simulink model "inverter_with_changing_VDC"  (R2013b)
settings: Solver=ode45  StartTime=0.0  StopTime=T  MaxStep=MaxStep  RelTol=RelTol
values from neighbouring files (symbols this model uses):
  a = b*(Cap*omega)    [it_generator.m]
  b = 0.0123    [it_generator.m]
  c3 = 1*(1+e+e3)    (= 1.11)    [initialization.m]
  Cap = 0.04    [initialization.m]
  ci = 1*(1-e)    (= 0.9)    [initialization.m]
  co = 1*(1+e)    (= 1.1)    [initialization.m]
  J = 2e4    (= 20000)    [initialization.m]
  L = 0.1    [initialization.m]
  R = 0.6    [initialization.m]
  rule = 1    [initialization.m]
  T = 8    [initialization.m]
  x0 = [iL0; vC0; p0;q0]    [initialization.m]
libraries: simulink x3
settings Model: Creator=Amy  LastModifiedBy=Amy

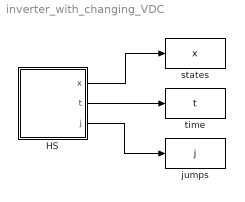
== system inverter_with_changing_VDC ==
  HS : Subsystem  LoadFcn=set_param(gcb,'LinkStatus','none')
      settings: CopyFcn=|
      | set_param(gcb,'LinkStatus','none'),
      | set_param(gcs, 'MaxStep', 'MaxStep', 'RelTol', 'RelTol','Stop time', 'T')
      mask Display:
      | image(imread('Hcal.jpg'))
      | %plot([5 20 20 5 5],[5 5 20 20 5])
      | %text(8,13,'HyEq_mdl')
      | port_label('output', 1, 'x')
      | port_label('output', 2, 't')
      | port_label('output', 3, 'j')
  jumps : ToWorkspace  VariableName=j  SampleTime=-1
  states : ToWorkspace  VariableName=x  SampleTime=-1
  time : ToWorkspace  VariableName=t  SampleTime=-1
  wires:
  HS/1(x) -> states/1
  HS/2(t) -> time/1
  HS/3(j) -> jumps/1

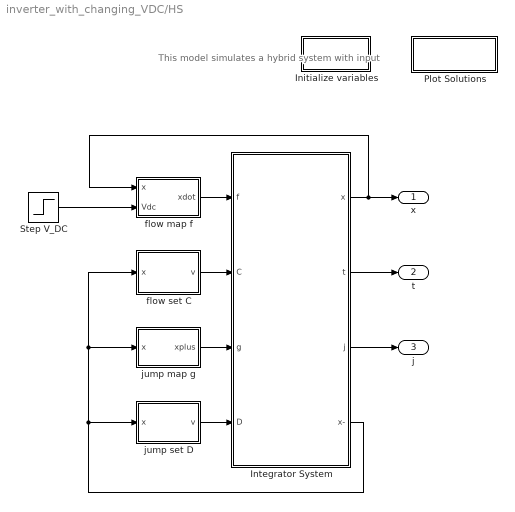
== system inverter_with_changing_VDC/HS ==
  note: This model simulates a hybrid system with input
  Initialize variables : Subsystem  Priority=-10
      settings: OpenFcn=|
      | try
      |      clearvars -except inifile pathfile_in pathfile_pos posfile
      |      cd(pathfile_in);
      |      eval(inifile);
      | catch
      |      [inifile,pathfile_in] = getInitializationfile;
      |      cd(pathfile_in);
      |      inifile = strrep(inifile,'.m','');
      |      eval(inifile);
      | end
      mask Display: disp('Double Click\n to Initialize')
  Integrator System : Subsystem  Priority=2  mask(Hybrid Integrator){T=T, J=J, x0=x0}
      mask prompts: T "Flow Horizon"; J "Jump Horizon"; x0 "Initial Condition"
      mask help:
      | This block integrates the state of the hybrid system defined by the flow map f (first input), the flow set C (second input), the jump map g (third input) and the jump set D (fourth input).
      | Starting from the initial condition x0 (last mask parameter), the system's state x evolves continuously within the set C, according to f(x,u), but is also subject to jumps within D, according to g(x,u).
      | The block also stops the simulation when the time t is greater than the flow horizon T (first mask parameter), or when the number of jumps j is greater than the jump horizon J (second mask parameter).
      | The outputs of the blocks are respectively x(t), t, j, x(t-).
      mask Help:
      | This block integrates the state of the hybrid system defined by the flow map f (first input), the flow set C (second input), the jump map g (third input) and the jump set D (fourth input).
      | <br>
      | Starting from the initial condition x0 (last mask parameter), the system's state x evolves continuously within the set C, according to f(x,u), but is also subject to jumps within D, according to g(x,u).
      | <br>
      | The block also stops the simulation when the time t is greater than the flow horizon T (first mask parameter), or when the number of jumps j is greater than the jump horizon J (second mask parameter).
      | <br>
      | The outputs of the blocks are respectively x(t), t, j, x(t-).
      | <br>
      | You can right click on the block and "Look under mask" to see what's inside the block.
      | Finally, refer to the manual (HybridSimulator_vXX.pdf) for more detailed information on how this hybrid simulator works.
  Plot Solutions : Subsystem
      settings: OpenFcn=|
      | try
      |      cd(pathfile_pos);
      |      eval(posfile);
      | catch
      |      [posfile,pathfile_pos] = getInitializationfile;
      |      cd(pathfile_pos);
      |      posfile = strrep(posfile,'.m','');
      |      eval(posfile);
      | end
      mask Display: disp('Double Click to\n Plot Solutions')
  Step V_DC : Step  Time=3  Before=5  After=7  SampleTime=0
  flow map f : MATLAB Function  TreatAsAtomicUnit=on
  flow set C : MATLAB Function  TreatAsAtomicUnit=on
  jump map g : MATLAB Function  Priority=2  TreatAsAtomicUnit=on
  jump set D : MATLAB Function  TreatAsAtomicUnit=on
  x : Outport
  t : Outport  Port=2
  j : Outport  Port=3
  wires:
  jump map g/1(xplus) -> Integrator System/3(g)
  jump set D/1(v) -> Integrator System/4(D)
  Integrator System/3(j) -> j/1
  Integrator System/2(t) -> t/1
  flow set C/1(v) -> Integrator System/2(C)
  Integrator System/1(x) -> flow map f/1(x), x/1
  Integrator System/4(x-) -> jump set D/1(x), jump map g/1(x), flow set C/1(x)
  flow map f/1(xdot) -> Integrator System/1(f)
  Step V_DC/1 -> flow map f/2(Vdc)

== system inverter_with_changing_VDC/HS/Initialize variables ==

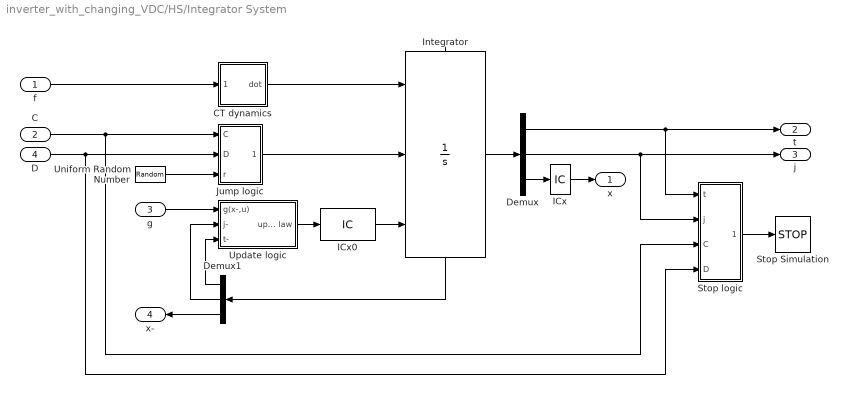
== system inverter_with_changing_VDC/HS/Integrator System ==
  f : Inport
  C : Inport  Port=2
  g : Inport  Port=3
  D : Inport  Port=4
  CT dynamics : Subsystem
  Demux : Demux  Outputs=[1 1 -1]
  Demux1 : Demux  Outputs=[1 1 -1]
  ICx : InitialCondition  Value=x0
  ICx0 : InitialCondition  Value=[0; 0; x0(:)]
  Integrator : Integrator  ExternalReset=level hold  InitialConditionSource=external  ShowStatePort=on  ZeroCross=off
  Jump logic : Subsystem
  Stop Simulation : Stop
  Stop logic : Subsystem
  Uniform Random Number : UniformRandomNumber  Minimum=0  Seed=abs(floor(100*rand))  SampleTime=0
  Update logic : Subsystem
  x : Outport
  t : Outport  Port=2
  j : Outport  Port=3
  x- : Outport  Port=4
  wires:
  ICx0/1 -> Integrator/3
  ICx/1 -> x/1
  Demux/3 -> ICx/1
  Integrator/State -> Demux1/1
  Demux/2 -> j/1, Stop logic/2(j)
  Demux/1 -> t/1, Stop logic/1(t)
  Update logic/1(update law) -> ICx0/1
  CT dynamics/1(dot) -> Integrator/1
  Stop logic/1(stop) -> Stop Simulation/1
  Integrator/1 -> Demux/1
  C/1 -> Stop logic/3(C), Jump logic/1(C)
  D/1 -> Stop logic/4(D), Jump logic/2(D)
  f/1 -> CT dynamics/1(f(x,u))
  Demux1/3 -> x-/1
  Jump logic/1(jump) -> Integrator/2
  Uniform Random Number/1 -> Jump logic/3(r)
  g/1 -> Update logic/1(g(x-,u))
  Demux1/1 -> Update logic/3(t-)
  Demux1/2 -> Update logic/2(j-)

== system inverter_with_changing_VDC/HS/Plot Solutions ==

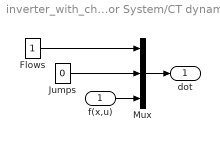
== system inverter_with_changing_VDC/HS/Integrator System/CT dynamics ==
  f(x,u) : Inport
  Flows : Constant
  Jumps : Constant  Value=0
  Mux : Mux  Inputs=[1 1 -1]
  dot : Outport
  wires:
  Jumps/1 -> Mux/2
  Flows/1 -> Mux/1
  Mux/1 -> dot/1
  f(x,u)/1 -> Mux/3

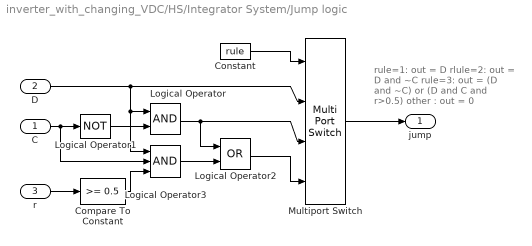
== system inverter_with_changing_VDC/HS/Integrator System/Jump logic ==
  note: rule=1:  out = D
      | rlule=2: out = D and ~C
      | rule=3:  out = (D and ~C)  or (D and C and r>0.5)
      | other :  out = 0
  C : Inport
  D : Inport  Port=2
  r : Inport  Port=3
  Compare To Constant : simulink/Logic and Bit Operations/Compare To Constant  relop=>=  const=0.5  OutDataTypeStr=uint8
  Constant : Constant  Value=rule
  Logical Operator : Logic  AllPortsSameDT=off  OutDataTypeStr=boolean
  Logical Operator1 : Logic  Operator=NOT  Inputs=1  AllPortsSameDT=off  OutDataTypeStr=boolean
  Logical Operator2 : Logic  Operator=OR  AllPortsSameDT=off  OutDataTypeStr=boolean
  Logical Operator3 : Logic  Inputs=3  AllPortsSameDT=off  OutDataTypeStr=boolean
  Multiport Switch : MultiPortSwitch
  jump : Outport
  wires:
  Constant/1 -> Multiport Switch/1
  D/1 -> Logical Operator3/1, Logical Operator/1, Multiport Switch/2
  r/1 -> Compare To Constant/1
  C/1 -> Logical Operator3/2, Logical Operator1/1
  Logical Operator1/1 -> Logical Operator/2
  Logical Operator/1 -> Multiport Switch/3, Logical Operator2/1
  Logical Operator2/1 -> Multiport Switch/4
  Multiport Switch/1 -> jump/1
  Compare To Constant/1 -> Logical Operator3/3
  Logical Operator3/1 -> Logical Operator2/2

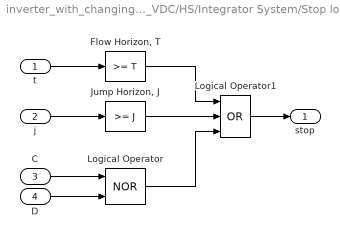
== system inverter_with_changing_VDC/HS/Integrator System/Stop logic ==
  t : Inport
  j : Inport  Port=2
  C : Inport  Port=3
  D : Inport  Port=4
  "Flow Horizon, T" : simulink/Logic and Bit Operations/Compare To Constant  relop=>=  const=T  OutDataTypeStr=uint8  ZeroCross=off
  "Jump Horizon, J" : simulink/Logic and Bit Operations/Compare To Constant  relop=>=  const=J  OutDataTypeStr=uint8  ZeroCross=off
  Logical Operator : Logic  Operator=NOR  AllPortsSameDT=off  OutDataTypeStr=boolean
  Logical Operator1 : Logic  Operator=OR  Inputs=3  AllPortsSameDT=off  OutDataTypeStr=boolean
  stop : Outport
  wires:
  "Flow Horizon, T"/1 -> Logical Operator1/1
  "Jump Horizon, J"/1 -> Logical Operator1/2
  Logical Operator/1 -> Logical Operator1/3
  D/1 -> Logical Operator/2
  t/1 -> "Flow Horizon, T"/1
  j/1 -> "Jump Horizon, J"/1
  C/1 -> Logical Operator/1
  Logical Operator1/1 -> stop/1

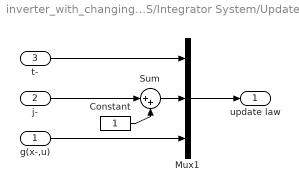
== system inverter_with_changing_VDC/HS/Integrator System/Update logic ==
  g(x-,u) : Inport
  j- : Inport  Port=2
  t- : Inport  Port=3
  Constant : Constant
  Mux1 : Mux  Inputs=[1 1 -1]
  Sum : Sum  Inputs=|++
  update law : Outport
  wires:
  Sum/1 -> Mux1/2
  Mux1/1 -> update law/1
  j-/1 -> Sum/1
  g(x-,u)/1 -> Mux1/3
  t-/1 -> Mux1/1
  Constant/1 -> Sum/2

== matlab function inverter_with_changing_VDC/HS/flow map f ==
  data: x input; xdot output; R parameter; L parameter; Cap parameter; Vdc input
function xdot = f(x, R, L, Cap, Vdc)
%%%%%%%%%%%%%%%%%%%%%%%%%%%%%%%%%%%%%%%%%%%%%%%%%%%%%%%%%%%%%%%%%%%%%%%%%%%
% Matlab M-file       
% Project: DC/AC inverter
%
% Name: f.m
%
% Description: Flow map
%
% Version: v1.8 lite
% Required files: - 
%%%%%%%%%%%%%%%%%%%%%%%%%%%%%%%%%%%%%%%%%%%%%%%%%%%%%%%%%%%%%%%%%%%%%%%%%%%
% states
  iL = x(1);
  vC = x(2);
  p = x(3);
  q = x(4);

% flow map
  iLdot = -R/L*iL - 1/L*vC + Vdc/L*q;
  vCdot = 1/Cap*iL;
  pdot = 0;
  qdot = 0;
  
xdot = [iLdot; vCdot; pdot; qdot];

== matlab function inverter_with_changing_VDC/HS/flow set C ==
  data: x input; v output; a parameter; b parameter; ci parameter; co parameter; c3 parameter; e1 parameter
function v  = C(x, a, b, ci, co, c3, e1) 
%%%%%%%%%%%%%%%%%%%%%%%%%%%%%%%%%%%%%%%%%%%%%%%%%%%%%%%%%%%%%%%%%%%%%%%%%%%
% Matlab M-file       
% Project: DC/AC inverter
%
% Name: C.m
%
% Description: Flow set
%
% Version: v1.8 
% Required files: - 
%%%%%%%%%%%%%%%%%%%%%%%%%%%%%%%%%%%%%%%%%%%%%%%%%%%%%%%%%%%%%%%%%%%%%%%%%%% 
% states
  iL = x(1);
  vC = x(2);
  p = x(3);
  q = x(4);

% useful expressions
  V = (iL/a)^2 + (vC/b)^2;
  qua = quadrant(iL, vC);  
  
% flow set
  if p == 1 
      if V >= ci && V <= co % Hs, Hfw flow
          v = 1;
      elseif q == -1 
          if iL <=0 &&  V <= ci % switch q accroding to Hfw 
              v = 1;
          elseif V >= co && V <= c3 && (qua == 1 || (qua == 4 && iL >= e1))
          % switch q accroding to Hfw
              v = 1;
          else
              v = 0;
          end
      elseif q == 1 
          if iL >=0 && V <= ci % switch q accroding to Hfw 
              v = 1;
          elseif V >= co && V <= c3 && (qua == 3 || (qua == 2 && iL <= -e1)) 
          % switch q accroding to Hfw 
              v = 1;
          else
              v = 0;
          end
      else
          v = 0;          
      end
  elseif p == 2
      if q == 0 && V >= co % Hs, Hg flow
          v = 1;
      elseif (q ~= 0) && V <= ci % Hs, Hg flow
          v = 1;
      else
          v = 0;
      end
  else 
      v = 0;
  end


% if V >= ci && V <= co && p == 1 % Hs, Hfw flow
%      v = 1;
%   elseif V <= ci && p == 1 && q == -1 && iL <=0 
%       % switch q accroding to Hfw 
%      v = 1;
%   elseif V >= co && V <= c3 && p == 1 && q == -1 && (qua == 1 || (qua == 4 && iL >= e1)) 
%       % switch q accroding to Hfw 
%      v = 1;
%   elseif V <= ci && p == 1 && q == 1 && iL >=0 
%       % switch q accroding to Hfw 
%      v = 1;
%   elseif V >= co && V <= c3 && p == 1 && q == 1 && (qua == 3 || (qua == 2 && iL <= -e1)) 
%       % switch q accroding to Hfw 
%      v = 1;
%      
%   elseif V >= co && p == 2 && q == 0 % Hs, Hg flow
%      v = 1;
%   elseif V <= ci && p == 2 && (q == 1 || q == -1) % Hs, Hg flow
%      v = 1;
%   else
%      v = 0;
%   end
% end

== matlab function inverter_with_changing_VDC/HS/jump map g ==
  data: x input; a parameter; b parameter; xplus output; co parameter; ci parameter; c3 parameter; e1 parameter
function xplus = g(x, a, b, co, ci, c3, e1)
%%%%%%%%%%%%%%%%%%%%%%%%%%%%%%%%%%%%%%%%%%%%%%%%%%%%%%%%%%%%%%%%%%%%%%%%%%%
% Matlab M-file       
% Project: DC/AC inverter
%
% Name: g.m
%
% Description: Jump map
%
% Version: v1.8 
% Required files: - 
%%%%%%%%%%%%%%%%%%%%%%%%%%%%%%%%%%%%%%%%%%%%%%%%%%%%%%%%%%%%%%%%%%%%%%%%%%%
% states
  iL = x(1);
  vC = x(2);
  p = x(3);
  q = x(4);  

% useful expressions
  V = (iL/a)^2 + (vC/b)^2;
  qua = quadrant(iL, vC);  
  
% jump map
  iLplus = iL;
  vCplus = vC;
  
  if p == 1
      if q ~= -1 && iL <=0 && V <= ci % switch q accroding to Hfw 
          pplus = p;
          qplus = -1;
      elseif q == 1 && V <= c3 && V >= co && (qua == 1 || (qua == 4 && iL >= e1)) 
      % switch q accroding to Hfw 
          pplus = p;
          qplus = -1;
      elseif V <= c3 && V >= co &&...
          ((qua == 4 && iL <= e1 && q == 1) || (qua == 2 && iL >= -e1 && q == -1))
      % switch q accroding to Hfw
          pplus = p;
          qplus = 0;
      elseif q ~= 1 && iL >=0 && V <= ci
      % switch q accroding to Hfw 
          pplus = p;
          qplus = 1;
      elseif q == -1 && V <= c3 && V >= co && (qua == 3 || (qua == 2 && iL <= -e1)) 
      % switch q accroding to Hfw 
          pplus = p;
          qplus = 1;
      else
          pplus = p;
          qplus = q;
      end
  elseif p == 2
      if  V >= ci && V <= co % Hs for switch controller
          pplus = 1;
          qplus = q;
      elseif q ~= 0 && V >= co% switch q accroding to Hg
          pplus = p;
          qplus = 0;
      elseif q == 0 && V <= ci% switch q accroding to Hg
          pplus = p;
          qplus = 1;   
      else
          pplus = p;
          qplus = q;
      end
  else
      pplus = p;
      qplus = q;
  end

% if V >= ci && V <= co && p == 2 % Hs for switch controller
%      pplus = 1;
%      qplus = q;
%   elseif V >= co && p == 2 && q ~= 0 % switch q accroding to Hg
%      pplus = p;
%      qplus = 0;
%   elseif V <= ci && p == 2 && q == 0 % switch q accroding to Hg
%      pplus = p;
%      qplus = 1;   
%   elseif V <= ci && p == 1 ...
%           && (q == 1 || q == 0) && iL <=0 
%       % switch q accroding to Hfw 
%      pplus = p;
%      qplus = -1;
%   elseif V <= c3 && V >= co && p == 1 && ...
%           q == 1 && (qua == 1 || (qua == 4 && iL >= e1)) 
%       % switch q accroding to Hfw 
%      pplus = p;
%      qplus = -1;
%   elseif V <= c3 && V >= co && p == 1 &&...
%           ((qua == 4 && iL <= e1 && q == 1) || (qua == 2 && iL >= -e1 && q == -1))
%       % switch q accroding to Hfw
%      pplus = p;
%      qplus = 0;
%   elseif V <= ci && p == 1 ...
%           && (q == -1 || q == 0) && iL >=0 
%       % switch q accroding to Hfw 
%      pplus = p;
%      qplus = 1;
%   elseif V <= c3 && V >= co && p == 1 && ...
%           q == -1 && (qua == 3 || (qua == 2 && iL <= -e1)) 
%       % switch q accroding to Hfw 
%      pplus = p;
%      qplus = 1;
%   else
%      pplus = p;
%      qplus = q;
%   end  
  
xplus = [iLplus; vCplus; pplus; qplus];
end

== matlab function inverter_with_changing_VDC/HS/jump set D ==
  data: x input; v output; co parameter; ci parameter; a parameter; b parameter; c3 parameter
function v  = D(x, co, ci, a, b, c3) 
%%%%%%%%%%%%%%%%%%%%%%%%%%%%%%%%%%%%%%%%%%%%%%%%%%%%%%%%%%%%%%%%%%%%%%%%%%%
% Matlab M-file       
% Project: DC/AC inverter
%
% Name: D.m
%
% Description: Jump set
%
% Version: v1.8 lite
% Required files: - 
%%%%%%%%%%%%%%%%%%%%%%%%%%%%%%%%%%%%%%%%%%%%%%%%%%%%%%%%%%%%%%%%%%%%%%%%%%%
% states
  iL = x(1);
  vC = x(2);
  p = x(3);
  q = x(4);

% useful expressions
  V = (iL/a)^2 + (vC/b)^2;
  qua = quadrant(iL, vC);  
  
% jump set
  if p == 1
      if q*iL <= 0 && V <= ci  % switch q accroding to Hfw
         v = 1;
      elseif q*iL >= 0 && V >= co && V <= c3 % switch q accroding to Hfw 
         v = 1;
      else
         v = 0;
      end
  elseif p == 2
      if q ~= 0 && V >= ci % switch q accroding to Hg
         v = 1;
      elseif q == 0 && V <= co % switch q accroding to Hg
         v = 1;
      else
         v = 0;
      end
  else 
      v = 0;
  end
  
end
